simulink model "inverter"  (R2021a)
settings: Solver=VariableStepAuto  StartTime=0.0  StopTime=20/f1  RelTol=1e-3
undefined symbols (not defined in the file): f1, ma, mf
libraries: spsDiodeLib x6, spsMosfetLib x6, spsVoltageMeasurementLib x4, spsSeriesRLCBranchLib x3, spsCurrentMeasurementLib x2, spsGroundLib x2, spsDCVoltageSourceLib x1, spsFirstOrderFilterLib x1, simulink x1, spspowerguiLib x1
settings Model: Creator=USUARIO  LastModifiedBy=USUARIO

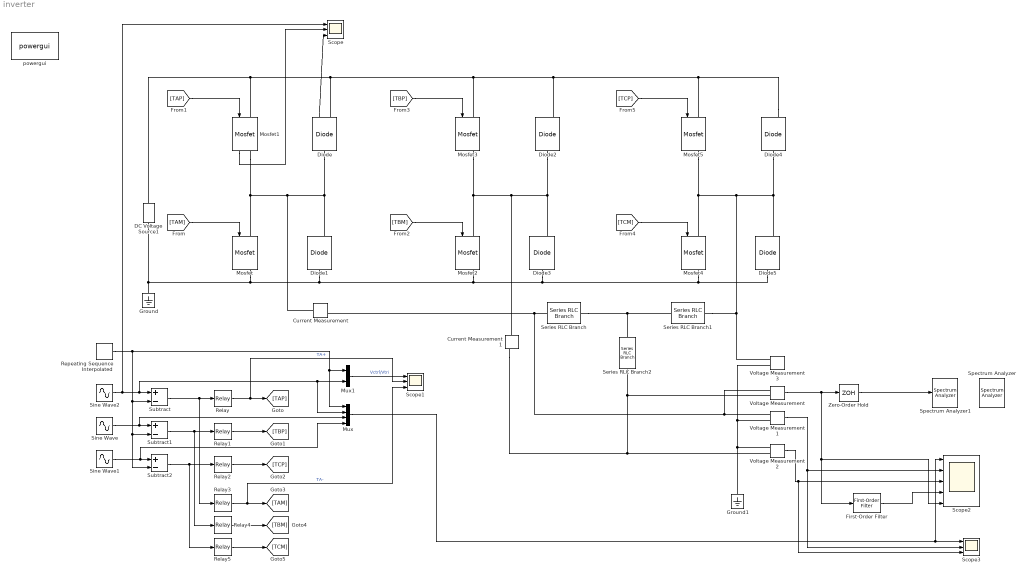
== system inverter ==
  Current Measurement : spsCurrentMeasurementLib/Current Measurement  PhasorSimulation=off  OutputType=Complex  PSBequivalent=0
  Current Measurement1 : spsCurrentMeasurementLib/Current Measurement  PhasorSimulation=off  OutputType=Complex  PSBequivalent=0
  DC Voltage Source1 : spsDCVoltageSourceLib/DC Voltage Source  Amplitude=311  Measurements=None
  Diode{,1..5} (6 alike) : spsDiodeLib/Diode  Ron=0.001  Lon=0  Vf=0.8  IC=0  UseSnubber=0  Rs=0  Cs=0  Measurements=on
  First-Order Filter : spsFirstOrderFilterLib/First-Order Filter  FilterType=Lowpass  Tc=1/(5*f1)  Ts=0  Initialize=on  Vac_Init=[0, 0, f1]  Vdc_Init=0  PlotResponse=off  FreqRange="[0,  200,  1]"
  Ground : spsGroundLib/Ground  LConnTagsString=a
  Ground1 : spsGroundLib/Ground  LConnTagsString=a
  Mosfet{,1..5} (6 alike) : spsMosfetLib/Mosfet  Ron=0.1  Lon=0  Rd=0.01  Vfd=0  IC=0  Rs=1e5  Cs=inf  Measurements=on
  Mux : Mux
  Mux1 : Mux  Inputs=2
  Relay : Relay
  Relay1 : Relay
  Relay2 : Relay
  Relay3 : Relay  OnOutputValue=0  OffOutputValue=1
  Relay4 : Relay  OnOutputValue=0  OffOutputValue=1
  Relay5 : Relay  OnOutputValue=0  OffOutputValue=1
  Repeating Sequence Interpolated : simulink/Sources/Repeating Sequence Interpolated  OutValues=[-1 1 -1].'  TimeValues=[0 1/(f1*mf) 2/(f1*mf)].'  LookUpMeth=Interpolation-Use End Values  tsamp=1/(50*mf*f1)  OutMin=[]  OutMax=[]  OutDataTypeStr=double  OutputDataTypeScalingMode=double  OutDataType=fixdt(0,8)  OutScaling=2^-10
  Scope : Scope  NumInputPorts=3
  Scope1 : Scope  NumInputPorts=3
  Scope2 : Scope  NumInputPorts=5
  Scope3 : Scope  NumInputPorts=3
  Series RLC Branch : spsSeriesRLCBranchLib/Series RLC Branch  LConnTagsString=__new0  RConnTagsString=__new0  BranchType=R  Resistance=20  Inductance=0  SetiL0=off  InitialCurrent=0  Capacitance=0  Setx0=off  InitialVoltage=0  Measurements=None
  Series RLC Branch1 : spsSeriesRLCBranchLib/Series RLC Branch  LConnTagsString=__new0  RConnTagsString=__new0  BranchType=R  Resistance=20  Inductance=0  SetiL0=off  InitialCurrent=0  Capacitance=0  Setx0=off  InitialVoltage=0  Measurements=None
  Series RLC Branch2 : spsSeriesRLCBranchLib/Series RLC Branch  LConnTagsString=__new0  RConnTagsString=__new0  BranchType=R  Resistance=20  Inductance=0  SetiL0=off  InitialCurrent=0  Capacitance=0  Setx0=off  InitialVoltage=0  Measurements=None
  Sine Wave : Sin  Amplitude=ma  Frequency=f1*2*pi  Phase=2*pi/3  SampleTime=0
  Sine Wave1 : Sin  Amplitude=ma  Frequency=f1*2*pi  Phase=4*pi/3  SampleTime=0
  Sine Wave2 : Sin  Amplitude=ma  Frequency=f1*2*pi  SampleTime=0
  Spectrum Analyzer : SpectrumAnalyzer
  Spectrum Analyzer1 : SpectrumAnalyzer
  Subtract : Sum  Inputs=+-
  Subtract1 : Sum  Inputs=+-
  Subtract2 : Sum  Inputs=+-
  Voltage Measurement{,1..3} (4 alike) : spsVoltageMeasurementLib/Voltage Measurement  PhasorSimulation=off  OutputType=Complex  PSBequivalent=0
  Zero-Order Hold : ZeroOrderHold  SampleTime=-1
  powergui : spspowerguiLib/powergui  Priority=1  SimulationMode=Continuous  SampleTime=50e-6  frequency=60  Iterations=50  frequencyindice=0  Pbase=100e6  ErrMax=1e-4  UnitsV=kV  UnitsW=MW  buscounter=0  FunctionMessages=off  echomessages=off  EnableUseOfTLC=off  CurrentSourceSwitches=off  DisableSnubberDevices=off  DisableRonSwitches=off  DisableVfSwitches=off  DisplayEquations=off  AutomaticDiscreteSolvers=off  SolverType=Tustin/Backward Euler (TBE)  Interpol=off  ExternalGateDelay=off  methode=off  Ts=100  x0status=blocks  SPID=on  SwTol=0  HookPort=off  NonlinearTolerance=1e-4  nMaxIteration=100  ContinueOnMaxIteration=off  RestoreLinks=warning  ResistiveCurrentMeasurement=off  Frange=[0:2:500]  Ylog=off  Xlog=on  ShowGrid=off  save=off  variable=ZData  structure=0  ZoomFFT=off  StartTime=0.0  cycles=1  DisplayStyle=1  fundamental=60  FreqAxis=off  MaxFrequency=1000  frequencyindicesteady=1  RmsSteady=1  display=off
  wires:
  Sine Wave/1 -> Mux/3, Subtract1/1
  Sine Wave1/1 -> Mux/4, Subtract2/1
  Repeating Sequence Interpolated/1 -> Mux/1, Mux1/1, Subtract2/2, Subtract1/2, Subtract/2
  Subtract/1 -> Relay3/1, Relay/1
  Subtract1/1 -> Relay4/1, Relay1/1
  Subtract2/1 -> Relay5/1, Relay2/1
  Relay/1 -> Scope1/2, [TAP]  "TA+"
  Relay1/1 -> [TBP]
  Relay2/1 -> [TCP]
  Relay5/1 -> [TCM]
  Relay4/1 -> [TBM]
  Relay3/1 -> Scope1/3, [TAM]  "TA-"
  [TAM] -> Mosfet/1
  [TAP] -> Mosfet1/1
  [TBM] -> Mosfet2/1
  [TBP] -> Mosfet3/1
  [TCP] -> Mosfet5/1
  [TCM] -> Mosfet4/1
  Diode/1 -> Scope/3
  Mosfet1/1 -> Scope/2
  Sine Wave2/1 -> Mux/2, Mux1/2, Subtract/1, Scope/1
  Mux1/1 -> Scope1/1  "Vctrl/Vtri"
  Zero-Order Hold/1 -> Spectrum Analyzer1/1
  Voltage Measurement/1 -> Scope2/5, First-Order Filter/1, Zero-Order Hold/1
  Mux/1 -> Scope2/1, Scope3/1
  Voltage Measurement1/1 -> Scope3/2, Scope2/2
  Voltage Measurement2/1 -> Scope3/3, Scope2/3
  First-Order Filter/1 -> Scope2/4
  connections:
  Mosfet1/RConn1 -- Current Measurement/LConn1 -- Diode/LConn1 -- Diode1/RConn1 -- Mosfet/LConn1
  Mosfet4/RConn1 -- DC Voltage Source1/LConn1 -- Ground/LConn1 -- Mosfet/RConn1 -- Diode1/LConn1 -- Mosfet2/RConn1 -- Diode3/LConn1 -- Diode5/LConn1
  Diode4/RConn1 -- Diode2/RConn1 -- Mosfet1/LConn1 -- DC Voltage Source1/RConn1 -- Diode/RConn1 -- Mosfet3/LConn1 -- Mosfet5/LConn1
  Mosfet3/RConn1 -- Current Measurement1/LConn1 -- Diode2/LConn1 -- Diode3/RConn1 -- Mosfet2/LConn1
  Mosfet5/RConn1 -- Voltage Measurement3/LConn1 -- Series RLC Branch1/RConn1 -- Diode4/LConn1 -- Diode5/RConn1 -- Mosfet4/LConn1
  Series RLC Branch/RConn1 -- Series RLC Branch1/LConn1 -- Series RLC Branch2/LConn1
  Series RLC Branch/LConn1 -- Voltage Measurement/LConn1 -- Voltage Measurement1/LConn1 -- Current Measurement/RConn1
  Current Measurement1/RConn1 -- Voltage Measurement/LConn2 -- Series RLC Branch2/RConn1 -- Voltage Measurement2/LConn2
  Voltage Measurement1/LConn2 -- Voltage Measurement3/LConn2 -- Ground1/LConn1 -- Voltage Measurement2/LConn1
